simulink model "omnimorph_controller_optim"  (R2023b)
settings: Solver=FixedStepAuto  StartTime=0.0  StopTime=inf  FixedStep=config.sim_var.time_step  RelTol=1e-3
libraries: genomix x5, robotcorelib x4, shareduavrstlib x1
settings Model: Creator=amr  LastModifiedBy=fiore
settings DataIOCC: ReturnWorkspaceOutputs=off
settings OptimizationCC: ReuseModelBlockBuffer=off
settings DebuggingCC: UnconnectedInputMsg=warning  UnconnectedOutputMsg=warning  UnconnectedLineMsg=warning  UnderSpecifiedDimensionMsg=warning
settings ModelReferenceCC: EnableRefExpFcnMdlSchedulingChecks=on
settings RTWCC: DLArmComputeVersion=19.05

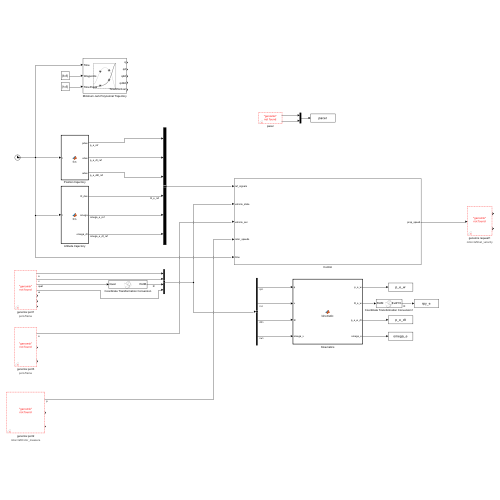
[thumbnail: Simulink's stored preview of the top-level diagram]
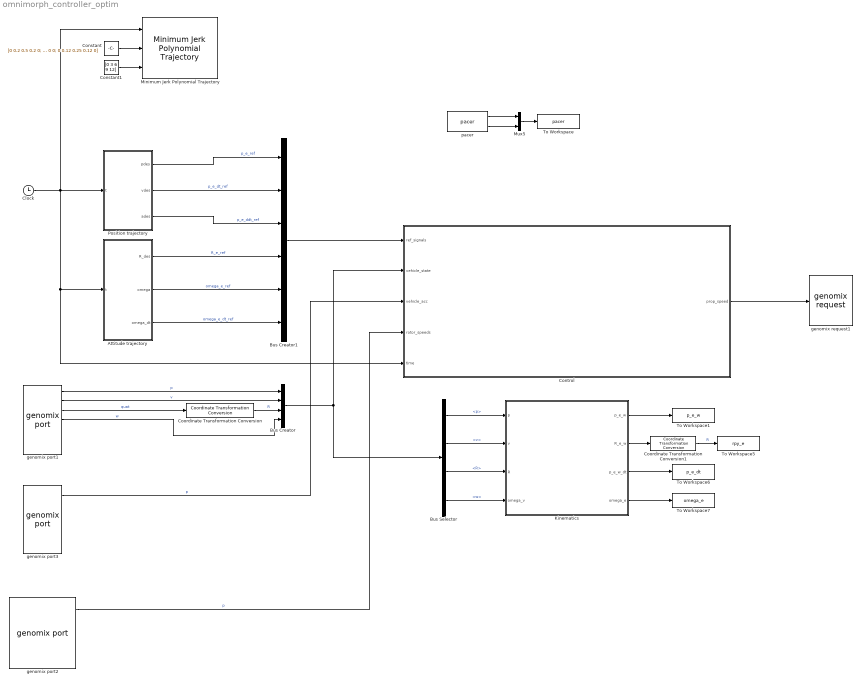
== system omnimorph_controller_optim ==
  Attitude trajectory : MATLAB Function  TreatAsAtomicUnit=on
  Bus Creator : BusCreator  Inputs=4
  Bus Creator1 : BusCreator  Inputs=6
  Bus Selector : BusSelector  OutputSignals=p,v,R,w
  Clock : Clock
  Constant : Constant  Value=[0 0.2 0.5 0.2 0; 0 0 0 0 0; 0 0.12 0.25 0.12 0]
  Constant1 : Constant  Value=[0 3 6 9 12]
  Control : Subsystem
  Coordinate Transformation Conversion : robotcorelib/Coordinate Transformation Conversion  InputRepresentation=Quaternion  InputEulerSequence=ZYX  ShowTrVecInputPort=on  OutputRepresentation=Rotation Matrix  OutputEulerSequence=ZYX  ShowTrVecOutputPort=on  SimulateUsing=Interpreted execution
  Coordinate Transformation Conversion1 : robotcorelib/Coordinate Transformation Conversion  InputRepresentation=Rotation Matrix  InputEulerSequence=ZYX  ShowTrVecInputPort=on  OutputRepresentation=Euler Angles  OutputEulerSequence=ZYX  ShowTrVecOutputPort=on  SimulateUsing=Interpreted execution
  Kinematics : MATLAB Function  TreatAsAtomicUnit=on
  Minimum Jerk Polynomial Trajectory : shareduavrstlib/Minimum Jerk Polynomial Trajectory  ShowBCInputPort=off  ShowPolynomialCoefs=off  ShowStatusOutputPort=off  TimeAllocation=off  TimeWeight=100  MinSegmentTime=0.1  MaxSegmentTime=1  MaxIteration=1500  MaxTime=10  SimulateUsing=Interpreted execution
      settings: LibrarySourceBlock=robotutilslib/Minimum Jerk Polynomial Trajectory
  Mux5 : Mux  Inputs=2
  Position trajectory : MATLAB Function  TreatAsAtomicUnit=on
  To Workspace : ToWorkspace  VariableName=pacer  SaveFormat=Timeseries  SampleTime=-1
  To Workspace1 : ToWorkspace  VariableName=p_e_w  SampleTime=-1
  To Workspace5 : ToWorkspace  VariableName=rpy_e  SampleTime=-1
  To Workspace6 : ToWorkspace  VariableName=p_e_dt  SampleTime=-1
  To Workspace7 : ToWorkspace  VariableName=omega_e  SampleTime=-1
  genomix port1 : genomix/genomix port  host=localhost  component=pom  port=frame  subport=robot  sigtype=value  timetype=periodic  period=config.sim_var.time_step  siglist="[{\"name\":\"frame.pos\",\"type\":\"value\",\"size\":3},{\"name\":\"frame.vel\",\"type\":\"value\",\"size\":3},{\"name\":\"frame.att\",\"type\":\"value\",\"size\":4},{\"name\":\"frame.avel\",\"type\":\"value\",\"size\":3},{\"name\":\"frame.intrinsic\",\"type\":\"value\",\"size\":1}]"
      settings: AttributesFormatString=pom/frame  SourceProductName=genomix
  genomix port2 : genomix/genomix port  host=localhost  component=rotorcraft  port=rotor_measure  sigtype=value  timetype=periodic  period=config.sim_var.time_step  siglist="[{\"name\":\"rotor_measure.rotor.velocity\",\"type\":\"value\",\"size\":8}]"
      settings: AttributesFormatString=rotorcraft/rotor_measure  SourceProductName=genomix
  genomix port3 : genomix/genomix port  host=localhost  component=pom  port=frame  subport=robot  sigtype=value  timetype=periodic  period=config.sim_var.time_step  siglist="[{\"name\":\"frame.acc\",\"type\":\"value\",\"size\":3}]"
      settings: AttributesFormatString=pom/frame  SourceProductName=genomix
  genomix request1 : genomix/genomix request  host=localhost  component=rotorcraft  port=set_velocity  sigtype=value  timetype=periodic  period=config.sim_var.time_step  siglist="[{\"name\":\"desired\",\"type\":\"value\",\"size\":8}]"
      settings: AttributesFormatString=rotorcraft/set_velocity  SourceProductName=genomix
  pacer : genomix/pacer  Priority=0  catchup=off
      settings: SourceProductName=genomix
  wires:
  Bus Creator1/1 -> Control/1(ref_signals)
  Clock/1 -> Minimum Jerk Polynomial Trajectory/1, Position trajectory/1(t), Control/5(time), Attitude trajectory/1(t)
  Attitude trajectory/1(R_des) -> Bus Creator1/4  "R_e_ref"
  Attitude trajectory/2(omega) -> Bus Creator1/5  "omega_e_ref"
  Attitude trajectory/3(omega_dt) -> Bus Creator1/6  "omega_e_dt_ref"
  genomix port1/1 -> Bus Creator/1  "p"
  genomix port1/2 -> Bus Creator/2  "v"
  genomix port1/4 -> Bus Creator/4  "w"
  genomix port1/3 -> Coordinate Transformation Conversion/1  "quat"
  Coordinate Transformation Conversion/1 -> Bus Creator/3  "R"
  Bus Creator/1 -> Control/2(vehicle_state), Bus Selector/1
  Control/1(prop_speed) -> genomix request1/1
  pacer/2 -> Mux5/2
  pacer/1 -> Mux5/1
  Mux5/1 -> To Workspace/1
  genomix port3/1 -> Control/3(vehicle_acc)  "p"
  genomix port2/1 -> Control/4(rotor_speeds)  "p"
  Kinematics/1(p_e_w) -> To Workspace1/1
  Kinematics/3(p_e_w_dt) -> To Workspace6/1
  Kinematics/4(omega_e) -> To Workspace7/1
  Coordinate Transformation Conversion1/1 -> To Workspace5/1  "R"
  Kinematics/2(R_e_w) -> Coordinate Transformation Conversion1/1
  Bus Selector/1 -> Kinematics/1(p)  "<p>"
  Bus Selector/2 -> Kinematics/2(v)  "<v>"
  Bus Selector/3 -> Kinematics/3(R)  "<R>"
  Bus Selector/4 -> Kinematics/4(omega_v)  "<w>"
  Constant1/1 -> Minimum Jerk Polynomial Trajectory/3
  Constant/1 -> Minimum Jerk Polynomial Trajectory/2
  Position trajectory/1(pdes) -> Bus Creator1/1  "p_e_ref"
  Position trajectory/2(vdes) -> Bus Creator1/2  "p_e_dt_ref"
  Position trajectory/3(ades) -> Bus Creator1/3  "p_e_ddt_ref"

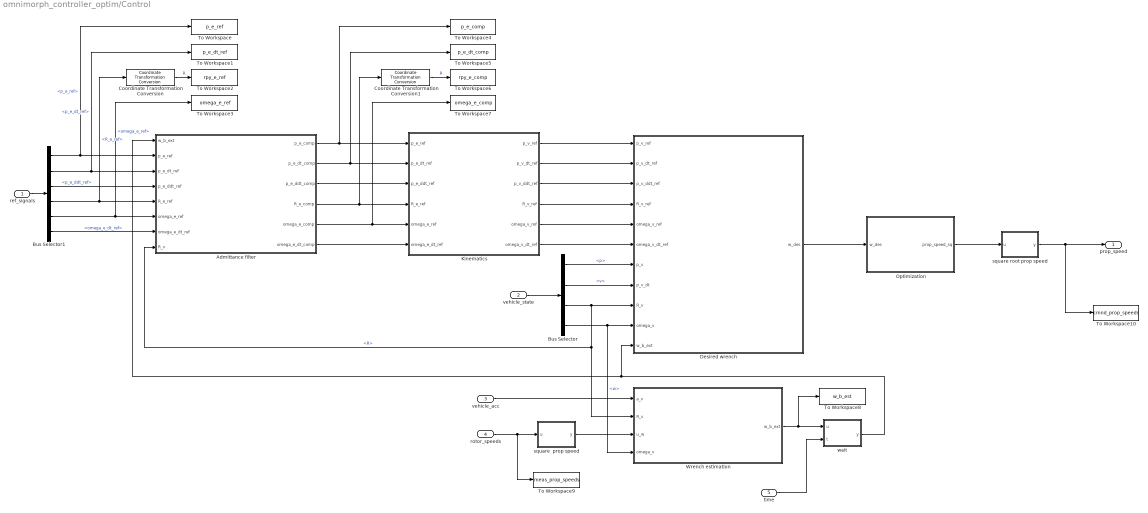
== system omnimorph_controller_optim/Control ==
  ref_signals : Inport
  vehicle_state : Inport  Port=2
  vehicle_acc : Inport  Port=3
  rotor_speeds : Inport  Port=4
  time : Inport  Port=5
  Admittance filter : Subsystem
  Bus Selector : BusSelector  OutputSignals=p,v,R,w
  Bus Selector1 : BusSelector  OutputSignals=p_e_ref,p_e_dt_ref,p_e_ddt_ref,R_e_ref,omega_e_ref,omega_e_dt_ref
  Coordinate Transformation Conversion : robotcorelib/Coordinate Transformation Conversion  InputRepresentation=Rotation Matrix  InputEulerSequence=ZYX  ShowTrVecInputPort=on  OutputRepresentation=Euler Angles  OutputEulerSequence=ZYX  ShowTrVecOutputPort=on  SimulateUsing=Interpreted execution
  Coordinate Transformation Conversion1 : robotcorelib/Coordinate Transformation Conversion  InputRepresentation=Rotation Matrix  InputEulerSequence=ZYX  ShowTrVecInputPort=on  OutputRepresentation=Euler Angles  OutputEulerSequence=ZYX  ShowTrVecOutputPort=on  SimulateUsing=Interpreted execution
  Desired wrench : MATLAB Function  TreatAsAtomicUnit=on
  Kinematics : MATLAB Function  TreatAsAtomicUnit=on
  Optimization : MATLAB Function  TreatAsAtomicUnit=on
  To Workspace : ToWorkspace  VariableName=p_e_ref  SampleTime=-1
  To Workspace1 : ToWorkspace  VariableName=p_e_dt_ref  SampleTime=-1
  To Workspace10 : ToWorkspace  VariableName=cmnd_prop_speeds  SampleTime=-1
  To Workspace2 : ToWorkspace  VariableName=rpy_e_ref  SampleTime=-1
  To Workspace3 : ToWorkspace  VariableName=omega_e_ref  SampleTime=-1
  To Workspace4 : ToWorkspace  VariableName=p_e_comp  SampleTime=-1
  To Workspace5 : ToWorkspace  VariableName=p_e_dt_comp  SampleTime=-1
  To Workspace6 : ToWorkspace  VariableName=rpy_e_comp  SampleTime=-1
  To Workspace7 : ToWorkspace  VariableName=omega_e_comp  SampleTime=-1
  To Workspace8 : ToWorkspace  VariableName=w_b_est  SampleTime=-1
  To Workspace9 : ToWorkspace  VariableName=meas_prop_speeds  SampleTime=-1
  Wrench estimation : Subsystem
  square  prop speed : MATLAB Function  TreatAsAtomicUnit=on
  square root prop speed : MATLAB Function  TreatAsAtomicUnit=on
  wait : MATLAB Function  TreatAsAtomicUnit=on
  prop_speed : Outport
  wires:
  Bus Selector/4 -> Desired wrench/10(omega_v), Wrench estimation/4(omega_v)  "<w>"
  ref_signals/1 -> Bus Selector1/1
  square root prop speed/1(y) -> To Workspace10/1, prop_speed/1
  Admittance filter/1(p_e_comp) -> To Workspace4/1, Kinematics/1(p_e_ref)
  Admittance filter/2(p_e_dt_comp) -> To Workspace5/1, Kinematics/2(p_e_dt_ref)
  Admittance filter/3(p_e_ddt_comp) -> Kinematics/3(p_e_ddt_ref)
  Admittance filter/6(omega_e_dt_comp) -> Kinematics/6(omega_e_dt_ref)
  Bus Selector1/6 -> Admittance filter/7(omega_e_dt_ref)  "<omega_e_dt_ref>"
  Bus Selector1/5 -> To Workspace3/1, Admittance filter/6(omega_e_ref)  "<omega_e_ref>"
  Bus Selector1/4 -> Admittance filter/5(R_e_ref), Coordinate Transformation Conversion/1  "<R_e_ref>"
  Bus Selector1/3 -> Admittance filter/4(p_e_ddt_ref)  "<p_e_ddt_ref>"
  Bus Selector1/2 -> To Workspace1/1, Admittance filter/3(p_e_dt_ref)  "<p_e_dt_ref>"
  Admittance filter/4(R_e_comp) -> Kinematics/4(R_e_ref), Coordinate Transformation Conversion1/1
  Kinematics/1(p_v_ref) -> Desired wrench/1(p_v_ref)
  Kinematics/2(p_v_dt_ref) -> Desired wrench/2(p_v_dt_ref)
  Kinematics/3(p_v_ddt_ref) -> Desired wrench/3(p_v_ddt_ref)
  Kinematics/5(omega_v_ref) -> Desired wrench/5(omega_v_ref)
  Kinematics/6(omega_v_dt_ref) -> Desired wrench/6(omega_v_dt_ref)
  Kinematics/4(R_v_ref) -> Desired wrench/4(R_v_ref)
  Admittance filter/5(omega_e_comp) -> Kinematics/5(omega_e_ref), To Workspace7/1
  Bus Selector/1 -> Desired wrench/7(p_v)  "<p>"
  Bus Selector/2 -> Desired wrench/8(p_v_dt)  "<v>"
  Bus Selector/3 -> Desired wrench/9(R_v), Wrench estimation/2(R_v), Admittance filter/8(R_v)  "<R>"
  Optimization/1(prop_speed_sq) -> square root prop speed/1(u)
  vehicle_state/1 -> Bus Selector/1
  vehicle_acc/1 -> Wrench estimation/1(a_v)
  rotor_speeds/1 -> To Workspace9/1, square  prop speed/1(u)
  square  prop speed/1(y) -> Wrench estimation/3(u_w)
  wait/1(y) -> Desired wrench/11(w_b_ext), Admittance filter/1(w_b_ext)
  time/1 -> wait/2(t)
  Bus Selector1/1 -> To Workspace/1, Admittance filter/2(p_e_ref)  "<p_e_ref>"
  Wrench estimation/1(w_b_ext) -> To Workspace8/1, wait/1(u)
  Coordinate Transformation Conversion/1 -> To Workspace2/1  "R"
  Coordinate Transformation Conversion1/1 -> To Workspace6/1  "R"
  Desired wrench/1(w_des) -> Optimization/1(w_des)

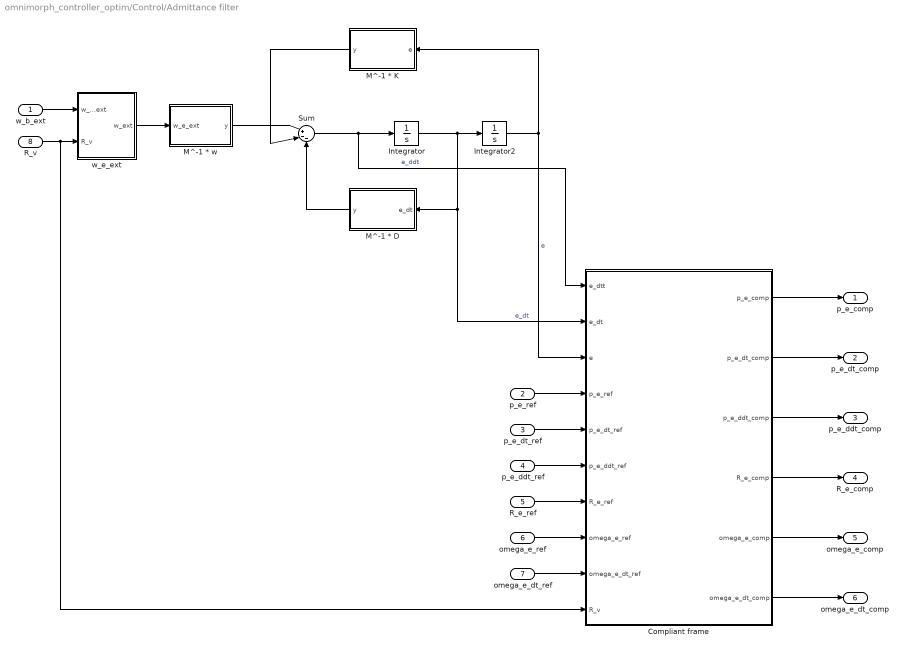
== system omnimorph_controller_optim/Control/Admittance filter ==
  w_b_ext : Inport
  p_e_ref : Inport  Port=2
  p_e_dt_ref : Inport  Port=3
  p_e_ddt_ref : Inport  Port=4
  R_e_ref : Inport  Port=5
  omega_e_ref : Inport  Port=6
  omega_e_dt_ref : Inport  Port=7
  R_v : Inport  Port=8
  Compliant frame : MATLAB Function  TreatAsAtomicUnit=on
  Integrator : Integrator
  Integrator2 : Integrator
  M^-1 * D : MATLAB Function  TreatAsAtomicUnit=on
  M^-1 * K : MATLAB Function  TreatAsAtomicUnit=on
  M^-1 * w : MATLAB Function  TreatAsAtomicUnit=on
  Sum : Sum  Inputs=|+--
  w_e_ext : MATLAB Function  TreatAsAtomicUnit=on
  p_e_comp : Outport
  p_e_dt_comp : Outport  Port=2
  p_e_ddt_comp : Outport  Port=3
  R_e_comp : Outport  Port=4
  omega_e_comp : Outport  Port=5
  omega_e_dt_comp : Outport  Port=6
  wires:
  Integrator/1 -> Compliant frame/2(e_dt), M^-1 * D/1(e_dt), Integrator2/1  "e_dt"
  Sum/1 -> Compliant frame/1(e_dtt), Integrator/1  "e_ddt"
  M^-1 * K/1(y) -> Sum/2
  Integrator2/1 -> Compliant frame/3(e), M^-1 * K/1(e)  "e"
  M^-1 * D/1(y) -> Sum/3
  p_e_ref/1 -> Compliant frame/4(p_e_ref)
  p_e_dt_ref/1 -> Compliant frame/5(p_e_dt_ref)
  p_e_ddt_ref/1 -> Compliant frame/6(p_e_ddt_ref)
  R_e_ref/1 -> Compliant frame/7(R_e_ref)
  omega_e_ref/1 -> Compliant frame/8(omega_e_ref)
  omega_e_dt_ref/1 -> Compliant frame/9(omega_e_dt_ref)
  Compliant frame/6(omega_e_dt_comp) -> omega_e_dt_comp/1
  Compliant frame/5(omega_e_comp) -> omega_e_comp/1
  Compliant frame/4(R_e_comp) -> R_e_comp/1
  Compliant frame/3(p_e_ddt_comp) -> p_e_ddt_comp/1
  Compliant frame/2(p_e_dt_comp) -> p_e_dt_comp/1
  Compliant frame/1(p_e_comp) -> p_e_comp/1
  M^-1 * w/1(y) -> Sum/1
  w_b_ext/1 -> w_e_ext/1(w_b_ext)
  w_e_ext/1(w_ext) -> M^-1 * w/1(w_e_ext)
  R_v/1 -> Compliant frame/10(R_v), w_e_ext/2(R_v)

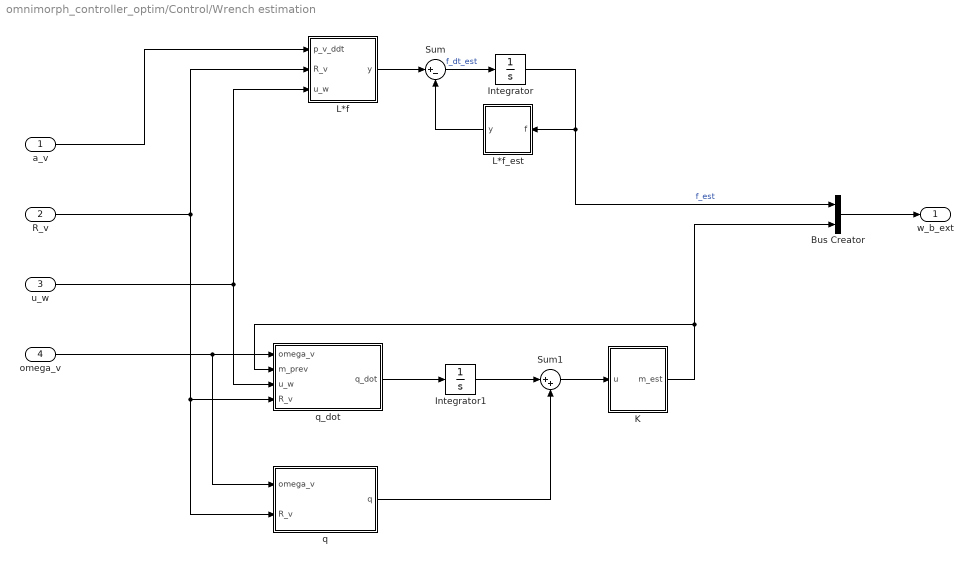
== system omnimorph_controller_optim/Control/Wrench estimation ==
  a_v : Inport
  R_v : Inport  Port=2
  u_w : Inport  Port=3
  omega_v : Inport  Port=4
  Bus Creator : BusCreator  Inputs=2
  Integrator : Integrator
  Integrator1 : Integrator
  K : MATLAB Function  TreatAsAtomicUnit=on
  L*f : MATLAB Function  TreatAsAtomicUnit=on
  L*f_est : MATLAB Function  TreatAsAtomicUnit=on
  Sum : Sum  Inputs=|+-
  Sum1 : Sum  Inputs=|++
  q : MATLAB Function  TreatAsAtomicUnit=on
  q_dot : MATLAB Function  TreatAsAtomicUnit=on
  w_b_ext : Outport
  wires:
  Sum/1 -> Integrator/1  "f_dt_est"
  Integrator/1 -> Bus Creator/1, L*f_est/1(f)  "f_est"
  L*f_est/1(y) -> Sum/2
  L*f/1(y) -> Sum/1
  R_v/1 -> q/2(R_v), q_dot/4(R_v), L*f/2(R_v)
  u_w/1 -> q_dot/3(u_w), L*f/3(u_w)
  omega_v/1 -> q/1(omega_v), q_dot/1(omega_v)
  a_v/1 -> L*f/1(p_v_ddt)
  Integrator1/1 -> Sum1/1
  q/1(q) -> Sum1/2
  Sum1/1 -> K/1(u)
  q_dot/1(q_dot) -> Integrator1/1
  Bus Creator/1 -> w_b_ext/1
  K/1(m_est) -> Bus Creator/2, q_dot/2(m_prev)

== matlab function omnimorph_controller_optim/Control/Admittance filter/M^-1 * w ==
  data: w_e_ext input; y output; config parameter
function y = fcn(w_e_ext,config)

M = config.cntrl_Admittance.params.M;
invM = diag([1/M(1,1);1/M(2,2);1/M(3,3);1/M(4,4);1/M(5,5);1/M(6,6)]);

y = invM*w_e_ext;

end

== matlab function omnimorph_controller_optim/Kinematics ==
  settings: updateMethod=DISCRETE
  data: p input; v input; R input; omega_v input; config parameter; p_e_w output; R_e_w output; p_e_w_dt output; omega_e output
function [p_e_w,R_e_w,p_e_w_dt,omega_e] = kinematic(p,v,R,omega_v,config)

p_e = config.uav_params.end_effector.p_e;
R_e = config.uav_params.end_effector.R_e;

p_e_w = p + R*p_e;
R_e_w = R*R_e;

omega_e = omega_v;
p_e_w_dt = v + R*skewMat(omega_v)*p_e;

end

== matlab function omnimorph_controller_optim/Control/Desired wrench ==
  settings: updateMethod=DISCRETE
  data: p_v_ref input; p_v_dt_ref input; p_v_ddt_ref input; R_v_ref input; omega_v_ref input; omega_v_dt_ref input; p_v input; p_v_dt input; R_v input; omega_v input; w_b_ext input; config parameter; w_des output
function w_des  = des_wrench(p_v_ref,p_v_dt_ref,p_v_ddt_ref, ...
                                          R_v_ref,omega_v_ref,omega_v_dt_ref,...
                                          p_v,p_v_dt,...
                                          R_v,omega_v,w_b_ext,config)

%% initializations
Kp = config.cntrl_opt.gains.Kp;
Kv = config.cntrl_opt.gains.Kv;
KR = config.cntrl_opt.gains.KR;
Kw = config.cntrl_opt.gains.Kw;

m = config.uav_params.mass;
J = config.uav_params.inertia;
J_inv = diag([1/J(1,1),1/J(2,2),1/J(3,3)]);
g = config.gravity;

omega_v_b = R_v.' * omega_v; % Body frame angular velocity

%% error signal computations 
ep =  p_v_ref - p_v;
ev = p_v_dt_ref - p_v_dt;

eR = vmap(R_v_ref,R_v);
ew = omega_v_ref - (R_v.')*R_v_ref*omega_v_b;
%ew = (omega_v_ref - omega_v);

%% compute w_des
f_ext = w_b_ext(1:3);
m_ext = w_b_ext(4:6);

f_des = R_v.' * (m*(g*[0;0;1] - (1/(m^2))*f_ext +  p_v_ddt_ref + Kv*ev + Kp*ep));
m_des = J * (J_inv*cross(omega_v_b,(J*omega_v_b)) - J_inv*m_ext + (omega_v_dt_ref + KR*eR + Kw*ew));

w_des = [f_des; m_des];

end

== matlab function omnimorph_controller_optim/Control/Optimization ==
  settings: updateMethod=DISCRETE
  data: w_des input; config parameter; prop_speed_sq output
function prop_speed_sq  = cntrl_alloc(w_des,config)

%% initializations
persistent prev_sol
A = config.uav_params.wrench_map;
w_p_min = config.uav_params.saturation.w_p_min;
w_p_max = config.uav_params.saturation.w_p_max;

%% Optimization
H = 2*eye(8);
f = zeros(8,1);
lb = -w_p_min^2 * ones(8,1);
ub = w_p_max^2 * ones(8,1);
opts = optimoptions('quadprog', 'Algorithm', 'active-set');
% x0 = zeros(8,1);

if isempty(prev_sol)
    prev_sol = zeros(8,1);
end

prop_speed_sq = quadprog(H, f, [], [], A, w_des, lb, ub, prev_sol, opts);

prev_sol = prop_speed_sq;

%prop_speed_sq = A \ w_des;
%prop_speed_sq = pinv(A)*w_des;

end

== matlab function omnimorph_controller_optim/Control/Kinematics ==
  settings: updateMethod=DISCRETE
  data: p_e_ref input; p_e_dt_ref input; p_e_ddt_ref input; R_e_ref input; omega_e_ref input; omega_e_dt_ref input; config parameter; p_v_ref output; p_v_dt_ref output; p_v_ddt_ref output; R_v_ref output; omega_v_ref output; omega_v_dt_ref output
function [p_v_ref,p_v_dt_ref,p_v_ddt_ref,R_v_ref,omega_v_ref,omega_v_dt_ref] = kinematic(p_e_ref,p_e_dt_ref,p_e_ddt_ref,R_e_ref,omega_e_ref,omega_e_dt_ref,config)

p_e = config.uav_params.end_effector.p_e;
R_e = config.uav_params.end_effector.R_e;

R_v_ref = R_e_ref*R_e.';
p_v_ref = p_e_ref - R_v_ref*p_e;

omega_v_ref = omega_e_ref;
p_v_dt_ref = p_e_dt_ref - R_v_ref*skewMat(omega_v_ref)*p_e;

omega_v_dt_ref = omega_e_dt_ref;
p_v_ddt_ref = p_e_ddt_ref - R_v_ref*skewMat(omega_v_dt_ref)*p_e - R_v_ref*skewMat(omega_v_ref)^2 *p_e;

end

== matlab function omnimorph_controller_optim/Control/Wrench estimation/L*f_est ==
  settings: updateMethod=DISCRETE
  data: f input; config parameter; y output
function y = fcn(f,config)

L = config.wrench_estimation.gains.L;
y = L*f;

end

== matlab function omnimorph_controller_optim/Control/Wrench estimation/L*f ==
  settings: updateMethod=DISCRETE
  data: p_v_ddt input; R_v input; u_w input; config parameter; y output
function y = fcn(p_v_ddt,R_v,u_w,config)

L = config.wrench_estimation.gains.L;
m = config.uav_params.mass;
g = config.gravity;
A = config.uav_params.wrench_map;

f = m*p_v_ddt + m*g*[0;0;1] - R_v*A(1:3,:)*u_w;

y = L*f;

end

== matlab function omnimorph_controller_optim/Control/Wrench estimation/q_dot ==
  settings: updateMethod=DISCRETE
  data: omega_v input; m_prev input; u_w input; R_v input; config parameter; q_dot output size=[3 1]
function q_dot = fcn(omega_v,m_prev,u_w,R_v,config)

A = config.uav_params.wrench_map;
J = config.uav_params.inertia;
omega_v_b = R_v'*omega_v; % Body frame angular velocity

q_dot = cross(omega_v_b,(J*omega_v_b)) - A(4:6,:)*u_w - m_prev;

end

== matlab function omnimorph_controller_optim/Control/Wrench estimation/q ==
  settings: updateMethod=DISCRETE
  data: omega_v input; R_v input; config parameter; q output
function q = fcn(omega_v,R_v,config)

J = config.uav_params.inertia;
omega_v_b = R_v'*omega_v; % Body frame angular velocity

% Assuming initial angular velocity is zero
q = J*omega_v_b;

end

== matlab function omnimorph_controller_optim/Control/Wrench estimation/K ==
  settings: updateMethod=DISCRETE
  data: u input; config parameter; m_est output
function m_est = fcn(u,config)

K = config.wrench_estimation.gains.K;
m_est = K*u;

end

== matlab function omnimorph_controller_optim/Control/Admittance filter/w_e_ext ==
  data: w_b_ext input; R_v input; w_ext output; config parameter
function w_ext = fcn(w_b_ext,R_v,config)

p_e = config.uav_params.end_effector.p_e;

H =  [eye(3),zeros(3);skewMat(R_v*p_e),eye(3)];
w_ext = H\[w_b_ext(1:3);R_v*w_b_ext(4:6)];

end

== matlab function omnimorph_controller_optim/Control/square root prop speed ==
  data: u input; y output
function y = fcn(u)
    y = [sign(u(1))*sqrt(abs(u(1)));sign(u(2))*sqrt(abs(u(2)));sign(u(3))*sqrt(abs(u(3)));
        sign(u(4))*sqrt(abs(u(4)));sign(u(5))*sqrt(abs(u(5)));sign(u(6))*sqrt(abs(u(6)));
        sign(u(7))*sqrt(abs(u(7)));sign(u(8))*sqrt(abs(u(8)))];
end

== matlab function omnimorph_controller_optim/Position trajectory ==
  data: t input; pdes output; vdes output; ades output; config parameter
function [pdes,vdes,ades] = fcn(t,config)

r = config.traj.params.radius;
f = config.traj.params.frequency;
z = 1;

% Circular trajectory
%if t<2
%    [pdes,vdes,ades] = circ_traj(t,0.5*t,f,0.5*t);
%    vdes(3) = 0.5;
%else
%    [pdes,vdes,ades] = circ_traj(t,r,f,z);
%end

% Peg-in-hole task
if t<2
    pdes = [0;0;0.5*t];
    vdes = [0;0;0.5];
    ades = [0;0;0];
elseif t>=2 && t<16.5
    pdes = [0.1*(t-2);0;0.99];
    vdes = [0.1;0;0];
    ades = [0;0;0];
else
    pdes = [(0.1*(16.5-2))-0.1*(t-16.5);0;0.99];
    vdes = [-0.1;0;0];
    ades = [0;0;0];    
end

% Sliding task
%if t<2
%    pdes = [0;0;0.5*t];
%    vdes = [0;0;0.5];
%    ades = [0;0;0];
%elseif t>=2 && t<14
%   pdes = [0.1*(t-2);0;1];
%   vdes = [0.1;0;0];
%   ades = [0;0;0]; 
%else
%   pdes = [1.2;0;1+0.1*(t-14)];
%   vdes = [0;0;0.1];
%   ades = [0;0;0]; 
%end

end

== matlab function omnimorph_controller_optim/Control/square  prop speed ==
  data: u input; y output
function y = fcn(u)
    y = [sign(u(1))*(abs(u(1))^2);sign(u(2))*(abs(u(2))^2);sign(u(3))*(abs(u(3))^2);
        sign(u(4))*(abs(u(4))^2);sign(u(5))*(abs(u(5))^2);sign(u(6))*(abs(u(6))^2);
        sign(u(7))*(abs(u(7))^2);sign(u(8))*(abs(u(8))^2)];
end

== matlab function omnimorph_controller_optim/Control/Admittance filter/M^-1 * K ==
  data: e input; y output; config parameter
function y = fcn(e,config)

K = config.cntrl_Admittance.params.K;
M = config.cntrl_Admittance.params.M;
%invM = diag([1/M(1,1);1/M(2,2);1/M(3,3)]);
invM = diag([1/M(1,1);1/M(2,2);1/M(3,3);1/M(4,4);1/M(5,5);1/M(6,6)]);

y = invM*K*e;

end

== matlab function omnimorph_controller_optim/Control/wait ==
  data: u input; y output; t input
function y = fcn(u,t)

    if t<1
        y = [0;0;0;0;0;0];
    else
        y = u;
    end

end

== matlab function omnimorph_controller_optim/Attitude trajectory ==
  data: R_des output; omega output; omega_dt output; t input; config parameter
function [R_des,omega,omega_dt] = fcn(t,config)

% Rotation about an axis
%if t<7
%    R_des = Rz(0)*Ry(0)*Rx(0);
%    omega = [0;0;0];
%    omega_dt = [0;0;0];
%elseif t>=7 && t<13
%    R_des = Rz(0)*Ry(0)*Rx(t-7);
%    omega = [1;0;0];
%    omega_dt = [0;0;0];
%else
%    R_des = Rz(0)*Ry(0)*Rx(0);
%    omega = [0;0;0];
%    omega_dt = [0;0;0];
%end

% Peg-in-hole task
if t<2
    R_des = Rz(0)*Ry(0)*Rx(0);
    omega = [0;0;0];
    omega_dt = [0;0;0];
else
    R_des = Rz(0)*Ry(pi/4)*Rx(0);
    omega = [0;0;0];
    omega_dt = [0;0;0];
end

%if t<2
%    R_des = Rz(0)*Ry(0)*Rx(0);
%    omega = [0;0;0];
%    omega_dt = [0;0;0];
%else
%    R_des = Rz(0)*Ry(t-2)*Rx(0);
%    omega = [0;1;0];
%    omega_dt = [0;0;0];
%end


% Sliding task
%R_des = Rz(0)*Ry(0)*Rx(0);
%omega = [0;0;0];
%omega_dt = [0;0;0];

end

== matlab function omnimorph_controller_optim/Control/Admittance filter/M^-1 * D ==
  data: e_dt input; y output; config parameter
function y = fcn(e_dt,config)

D = config.cntrl_Admittance.params.D;
M = config.cntrl_Admittance.params.M;
%invM = diag([1/M(1,1);1/M(2,2);1/M(3,3)]);
invM = diag([1/M(1,1);1/M(2,2);1/M(3,3);1/M(4,4);1/M(5,5);1/M(6,6)]);

y = invM*D*e_dt;

end

== matlab function omnimorph_controller_optim/Control/Admittance filter/Compliant frame ==
  data: e_dtt input; e_dt input; e input; p_e_ref input; p_e_dt_ref input; p_e_ddt_ref input; R_e_ref input; omega_e_ref input; omega_e_dt_ref input; R_v input; p_e_comp output; config parameter; p_e_dt_comp output; p_e_ddt_comp output; R_e_comp output; omega_e_comp output; omega_e_dt_comp output
function [p_e_comp,p_e_dt_comp,p_e_ddt_comp,R_e_comp,omega_e_comp,omega_e_dt_comp] = fcn(e_dtt,e_dt,e,p_e_ref,p_e_dt_ref,p_e_ddt_ref, ...
                                                                                 R_e_ref,omega_e_ref,omega_e_dt_ref,R_v,config)
p_e_comp = p_e_ref + e(1:3);
p_e_dt_comp = p_e_dt_ref + e_dt(1:3);
p_e_ddt_comp = p_e_ddt_ref + e_dtt(1:3);

%R_e_comp = R_e_ref*(skewMat(e(4:6)) + eye(3));
R_e_comp = R_e_ref*(eye(3) - skewMat(e(4:6))); % Simply invert error
%vector??
R_e_comp = (skewMat(e(4:6)) + eye(3))*R_e_ref;
omega_e_comp = R_v'*(R_v*omega_e_ref + e_dt(4:6));
omega_e_dt_comp = R_v'*(R_v*omega_e_dt_ref + e_dtt(4:6));

end
